simulink model "my_robot_1"  (R2013a)
settings: Solver=ode4  StartTime=0.0  StopTime=T  FixedStep=1/fs  RelTol=1e-3
values from neighbouring files (symbols this model uses):
  Kp = eye(robot.n) * k * (pi*fs)^2    [Ejercicio1.m]    (also in Ejercicio2.m = Kp/Wall.Ke)
  Kv = 2*sqrt(Kp)    [Ejercicio1.m]    (also in Ejercicio2.m)
  thetai = robot.ikine(Ti, [0, pi/2], [1 1 0 0 0 0])    [Ejercicio1.m]    (also in Ejercicio2.m; Ejercicio3.m)
settings Model: Creator=Juan Pablo  LastModifiedBy=root
settings DataIOCC: ExternalInput=[t, xSetpoint]  LimitDataPoints=off  LoadExternalInput=on  SaveTime=off  OutputSaveName=q, x

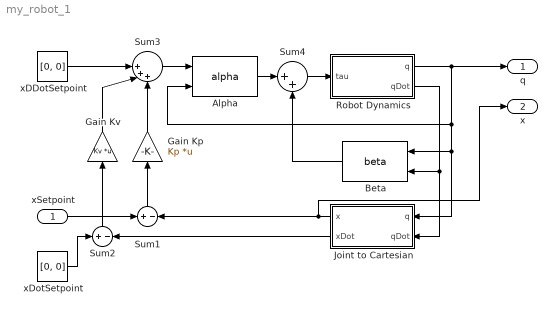
== system my_robot_1 ==
  xSetpoint : Inport  PortDimensions=2
  Alpha : M-S-Function  FunctionName=alpha  Parameters=robot
  Beta : M-S-Function  FunctionName=beta  Parameters=robot
  Gain Kp : Gain  Gain=Kp  Multiplication=Matrix(K*u)
  Gain Kv : Gain  Gain=Kv  Multiplication=Matrix(K*u)
  Joint to Cartesian : Subsystem
  Robot Dynamics : Subsystem
  Sum1 : Sum  Inputs=+|-
  Sum2 : Sum  Inputs=+|-
  Sum3 : Sum  Inputs=||+++
  Sum4 : Sum  Inputs=|++
  xDDotSetpoint : Constant  Value=[0, 0]
  xDotSetpoint : Constant  Value=[0, 0]
  q : Outport
  x : Outport  Port=2
  wires:
  Robot Dynamics/1(q) -> q/1, Alpha/2, Joint to Cartesian/1(q), Beta/1
  Robot Dynamics/2(qDot) -> Joint to Cartesian/2(qDot), Beta/2
  xSetpoint/1 -> Sum1/1
  Sum2/1 -> Gain Kv/1
  Sum1/1 -> Gain Kp/1
  Alpha/1 -> Sum4/1
  Sum3/1 -> Alpha/1
  xDDotSetpoint/1 -> Sum3/1
  xDotSetpoint/1 -> Sum2/1
  Gain Kp/1 -> Sum3/3
  Joint to Cartesian/1(x) -> x/1, Sum1/2
  Joint to Cartesian/2(xDot) -> Sum2/2
  Sum4/1 -> Robot Dynamics/1(tau)
  Beta/1 -> Sum4/2
  Gain Kv/1 -> Sum3/2

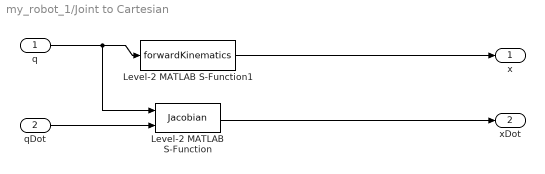
== system my_robot_1/Joint to Cartesian ==
  q : Inport
  qDot : Inport  Port=2
  Level-2 MATLAB S-Function : M-S-Function  FunctionName=Jacobian  Parameters=robot
  Level-2 MATLAB S-Function1 : M-S-Function  FunctionName=forwardKinematics  Parameters=robot
  x : Outport
  xDot : Outport  Port=2
  wires:
  q/1 -> Level-2 MATLAB S-Function1/1, Level-2 MATLAB S-Function/1
  qDot/1 -> Level-2 MATLAB S-Function/2
  Level-2 MATLAB S-Function/1 -> xDot/1
  Level-2 MATLAB S-Function1/1 -> x/1

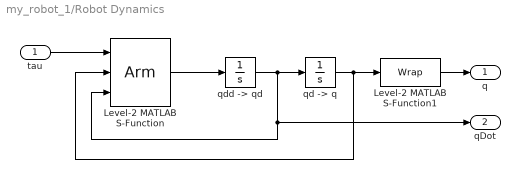
== system my_robot_1/Robot Dynamics ==
  tau : Inport
  Level-2 MATLAB S-Function : M-S-Function  FunctionName=Arm  Parameters=probot
  Level-2 MATLAB S-Function1 : M-S-Function  FunctionName=Wrap  Parameters=robot
  "qd -> q" : Integrator  InitialCondition=thetai
  "qdd -> qd" : Integrator
  q : Outport
  qDot : Outport  Port=2
  wires:
  Level-2 MATLAB S-Function/1 -> "qdd -> qd"/1
  "qdd -> qd"/1 -> Level-2 MATLAB S-Function/3, qDot/1, "qd -> q"/1
  "qd -> q"/1 -> Level-2 MATLAB S-Function/2, Level-2 MATLAB S-Function1/1
  tau/1 -> Level-2 MATLAB S-Function/1
  Level-2 MATLAB S-Function1/1 -> q/1
